simulink model "sa_aproksimacijom"  (Simulink 6.0)
settings: Solver=ode3  StartTime=0.0  StopTime=20  FixedStep=0.001  RelTol=1e-3
values from neighbouring files (symbols this model uses):
  a = input('Unesi vrijednost a:' )    [Kod.m]
  alfa0 = input('Unesi pocetnu vrijednost ugla alfa:' )    [Kod.m]
  beta0 = input('Unesi pocetnu vrijednost ugla beta:')    [Kod.m]
  g = 9.80665    [Kod.m]
  gama0 = input('Unesi pocetnu vrijednost ugla gama:')    [Kod.m]
  k = input('Unesi krutost opruge k:' )    [Kod.m]
  m = input('Unesi masu tijela:')    [Kod.m]
settings Model: LastModifiedBy=Administrator

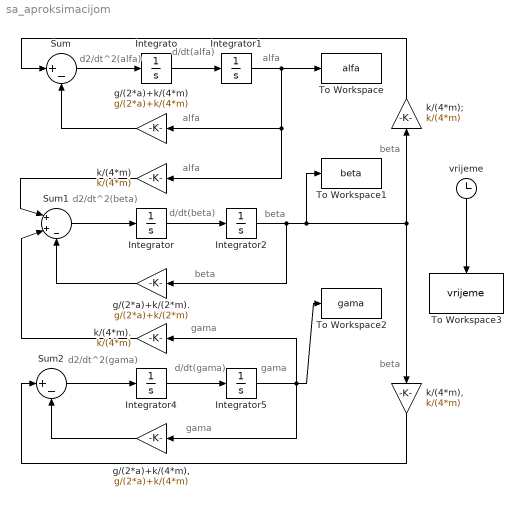
== system sa_aproksimacijom ==
  note: d2/dt^2(alfa)
  note: d/dt(alfa)
  note: alfa
  note: d2/dt^2(beta)
  note: d2/dt^2(gama)
  note: d/dt(beta)
  note: d/dt(gama)
  note: beta
  note: gama
  note: alfa
  note: alfa
  note: gama
  note: gama
  note: beta
  note: beta
  note: beta
  Integrato : Integrator
  Integrator : Integrator
  Integrator1 : Integrator  InitialCondition=alfa0
  Integrator2 : Integrator  InitialCondition=beta0
  Integrator4 : Integrator
  Integrator5 : Integrator  InitialCondition=gama0
  Sum : Sum  Inputs=|+-
  Sum1 : Sum  Inputs=|++-
  Sum2 : Sum  Inputs=|+-
  To Workspace : ToWorkspace  VariableName=alfa  SampleTime=-1  SaveFormat=Array
  To Workspace1 : ToWorkspace  VariableName=beta  SampleTime=-1  SaveFormat=Array
  To Workspace2 : ToWorkspace  VariableName=gama  SampleTime=-1  SaveFormat=Array
  To Workspace3 : ToWorkspace  VariableName=vrijeme  SampleTime=-1  SaveFormat=Array
      settings: Orientation=down
  g/(2*a)+k/(2*m). : Gain  Orientation=left  Gain=g/(2*a)+k/(2*m)
  g/(2*a)+k/(4*m) : Gain  Orientation=left  Gain=g/(2*a)+k/(4*m)
  g/(2*a)+k/(4*m), : Gain  Orientation=left  Gain=g/(2*a)+k/(4*m)
  k/(4*m) : Gain  Orientation=left  Gain=k/(4*m)
  k/(4*m), : Gain  Orientation=down  Gain=k/(4*m)
  k/(4*m). : Gain  Orientation=left  Gain=k/(4*m)
  k/(4*m); : Gain  Orientation=up  Gain=k/(4*m)
  vrijeme : Clock
      settings: Orientation=down  Decimation=10
  wires:
  Integrato/1 -> Integrator1/1
  Integrator1/1 -> g/(2*a)+k/(4*m)/1, k/(4*m)/1, To Workspace/1
  g/(2*a)+k/(4*m)/1 -> Sum/2
  Sum/1 -> Integrato/1
  Integrator/1 -> Integrator2/1
  Sum1/1 -> Integrator/1
  Integrator2/1 -> g/(2*a)+k/(2*m)./1, To Workspace1/1, k/(4*m);/1, k/(4*m),/1
  g/(2*a)+k/(2*m)./1 -> Sum1/3
  k/(4*m)/1 -> Sum1/1
  k/(4*m)./1 -> Sum1/2
  k/(4*m);/1 -> Sum/1
  Integrator4/1 -> Integrator5/1
  Sum2/1 -> Integrator4/1
  Integrator5/1 -> k/(4*m)./1, g/(2*a)+k/(4*m),/1, To Workspace2/1
  g/(2*a)+k/(4*m),/1 -> Sum2/2
  k/(4*m),/1 -> Sum2/1
  vrijeme/1 -> To Workspace3/1
